simulink model "modeloSS_yama_LQI"  (R2016b)
settings: Solver=FixedStepDiscrete  StartTime=0.0  StopTime=20  FixedStep=0.001  RelTol=1e-3  EnableMultiTasking=on
values from neighbouring files (symbols this model uses):
  K_lqi = lqi(manolito,Q,R,N)    [marcelino_Lineal_LQI.m]
  Kb = 0.468    [Jacobian_marcelino.m]
  Kt = 0.317    [Jacobian_marcelino.m]    (also in Jacobian_marcelinoB.m)
  Rm = 6.69    [Jacobian_marcelino.m]    (also in Jacobian_marcelinoB.m)
undefined symbols (not defined in the file or in its folder): Cm, Cw, DiscIntNeverNeededParam, Jm, Jw, Lm, n
libraries: simulink x1
settings Model: Creator=FranRuzafa  LastModifiedBy=Miguel
settings OptimizationCC: LifeSpan=inf
settings DebuggingCC: SFUnexpectedBacktrackingDiag=warning  SFNoUnconditionalDefaultTransitionDiag=warning  SFExecutionAtInitializationDiag=none
settings GRTTargetCC: TargetLangStandard=C89/C90 (ANSI)  GeneratePreprocessorConditionals=Disable all
settings ConfigComp: CovMetricSettings=dw  CovHtmlReporting=on  CovSaveCumulativeToWorkspaceVar=on  CovSaveSingleToWorkspaceVar=on  CovExternalEMLEnable=off

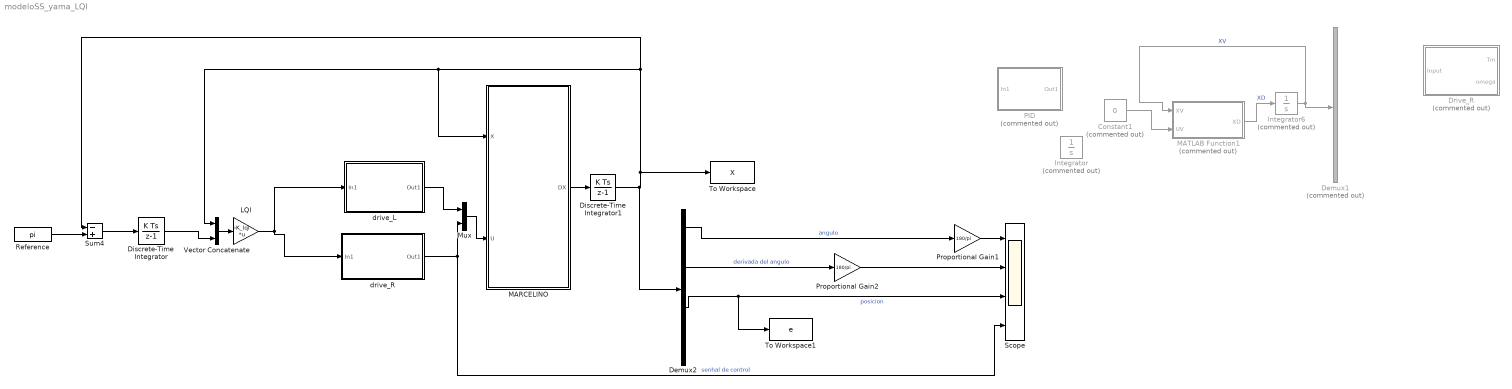
== system modeloSS_yama_LQI ==
  Constant1 : Constant  Commented=on  Value=0
  Demux1 : Demux  Commented=on
  Demux2 : Demux
  Discrete-Time Integrator : DiscreteIntegrator  InitialConditionSetting=State (most efficient)  SampleTime=-1  ICPrevOutput=DiscIntNeverNeededParam  ICPrevScaledInput=DiscIntNeverNeededParam
  Discrete-Time Integrator1 : DiscreteIntegrator  InitialCondition=[pi+0.2,0,0,0]  InitialConditionSetting=State (most efficient)  SampleTime=-1  ICPrevOutput=DiscIntNeverNeededParam  ICPrevScaledInput=DiscIntNeverNeededParam
  Drive_R : Subsystem  Commented=on
  Integrator : Integrator  Commented=on  InitialCondition=[pi+0.2,0,0,0]
  Integrator6 : Integrator  Commented=on  InitialCondition=[0;0;0.1;0]
  "LQI " : Gain  Gain=-K_lqi  Multiplication=Matrix(K*u)  SaturateOnIntegerOverflow=on  OutDataTypeStr=Inherit: Same as input  ParamDataTypeStr=Inherit: Same as input
  MARCELINO : MATLAB Function  TreatAsAtomicUnit=on
  MATLAB Function1 : MATLAB Function  Commented=on  TreatAsAtomicUnit=on
  Mux : Mux  Inputs=2
  PID : Subsystem  Commented=on
  Proportional Gain1 : Gain  Gain=180/pi  SaturateOnIntegerOverflow=on  OutDataTypeStr=Inherit: Same as input  ParamDataTypeStr=Inherit: Same as input
  Proportional Gain2 : Gain  Gain=180/pi  SaturateOnIntegerOverflow=on  OutDataTypeStr=Inherit: Same as input  ParamDataTypeStr=Inherit: Same as input
  Reference : Constant  Value=pi
  Scope : Scope  NumInputPorts=4
  Sum4 : Sum  Inputs=-+  SaturateOnIntegerOverflow=on  InputSameDT=on  OutDataTypeStr=Inherit: Same as first input
  To Workspace : ToWorkspace  VariableName=X  SampleTime=-1
      settings: Save2DSignal=2-D array (concatenate along first dimension)
  To Workspace1 : ToWorkspace  VariableName=e  SampleTime=-1
      settings: Save2DSignal=2-D array (concatenate along first dimension)
  Vector Concatenate : Concatenate
  drive_L : Subsystem
  "drive_R " : Subsystem
  wires:
  MARCELINO/1(DX) -> Discrete-Time Integrator1/1
  MATLAB Function1/1(XD) -> Integrator6/1  "XD"
  Integrator6/1 -> Demux1/1, MATLAB Function1/1(XV)  "XV"
  Constant1/1 -> MATLAB Function1/2(UV)
  Discrete-Time Integrator1/1 -> Demux2/1, Sum4/1, MARCELINO/1(X), Vector Concatenate/1, To Workspace/1
  Demux2/1 -> Proportional Gain1/1  "angulo"
  Reference/1 -> Sum4/2
  Proportional Gain1/1 -> Scope/1
  Sum4/1 -> Discrete-Time Integrator/1
  "drive_R "/1(Out1) -> Mux/2, Scope/4  "senhal de control"
  "LQI "/1 -> "drive_R "/1(In1), drive_L/1(In1)
  drive_L/1(Out1) -> Mux/1
  Mux/1 -> MARCELINO/2(U)
  Discrete-Time Integrator/1 -> Vector Concatenate/2
  Vector Concatenate/1 -> "LQI "/1
  Demux2/3 -> To Workspace1/1, Scope/3  "posicion"
  Demux2/2 -> Proportional Gain2/1  "derivada del angulo"
  Proportional Gain2/1 -> Scope/2

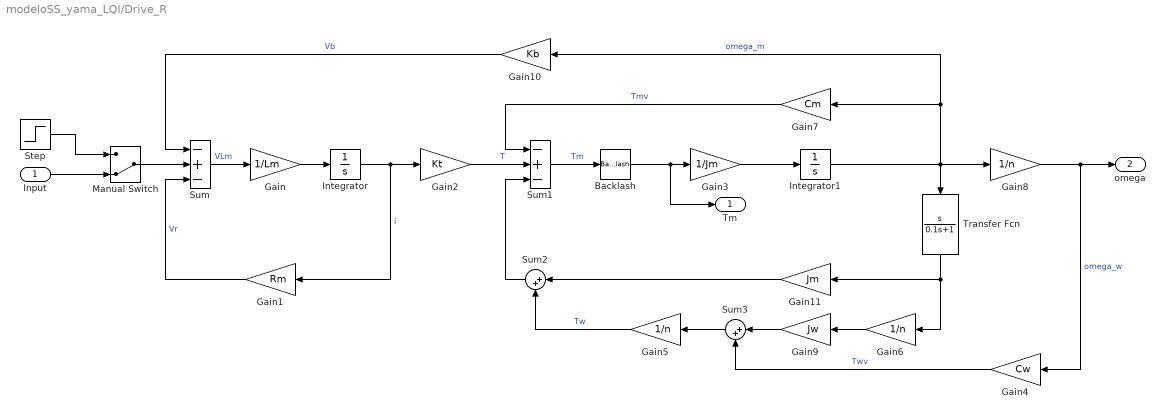
== system modeloSS_yama_LQI/Drive_R ==
  Input : Inport
  Backlash : Backlash  BacklashWidth=0.05
  Gain : Gain  Gain=1/Lm
  Gain1 : Gain  Gain=Rm
  Gain10 : Gain  Gain=Kb
  Gain11 : Gain  Gain=Jm
  Gain2 : Gain  Gain=Kt
  Gain3 : Gain  Gain=1/Jm
  Gain4 : Gain  Gain=Cw
  Gain5 : Gain  Gain=1/n
  Gain6 : Gain  Gain=1/n
  Gain7 : Gain  Gain=Cm
  Gain8 : Gain  Gain=1/n
  Gain9 : Gain  Gain=Jw
  Integrator : Integrator
  Integrator1 : Integrator
  Manual Switch : ManualSwitch  CurrentSetting=0
  Step : Step  After=9  SampleTime=0
  Sum : Sum  Inputs=-+-
  Sum1 : Sum  Inputs=-+-
  Sum2 : Sum  Inputs=|++
  Sum3 : Sum  Inputs=|++
  Transfer Fcn : TransferFcn  Numerator=[1 0]  Denominator=[0.1 1]
  Tm : Outport
  omega : Outport  Port=2
  wires:
  Sum/1 -> Gain/1  "VLm"
  Gain/1 -> Integrator/1
  Integrator/1 -> Gain2/1, Gain1/1  "i"
  Gain1/1 -> Sum/3  "Vr"
  Gain2/1 -> Sum1/2  "T"
  Sum1/1 -> Backlash/1  "Tm"
  Gain3/1 -> Integrator1/1
  Gain7/1 -> Sum1/1  "Tmv"
  Integrator1/1 -> Gain10/1, Gain7/1, Gain8/1, Transfer Fcn/1  "omega_m"
  Gain10/1 -> Sum/1  "Vb"
  Gain6/1 -> Gain9/1
  Sum3/1 -> Gain5/1
  Transfer Fcn/1 -> Gain6/1, Gain11/1
  Gain4/1 -> Sum3/2  "Twv"
  Gain9/1 -> Sum3/1
  Gain8/1 -> omega/1, Gain4/1  "omega_w"
  Manual Switch/1 -> Sum/2
  Input/1 -> Manual Switch/2
  Step/1 -> Manual Switch/1
  Sum2/1 -> Sum1/3
  Gain5/1 -> Sum2/2  "Tw"
  Gain11/1 -> Sum2/1
  Backlash/1 -> Gain3/1, Tm/1

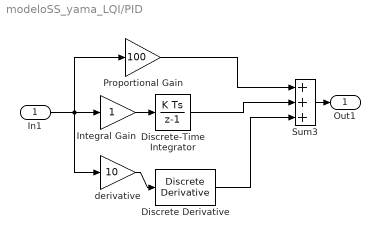
== system modeloSS_yama_LQI/PID ==
  In1 : Inport
  Discrete Derivative : simulink/Discrete/Discrete Derivative  gainval=1.0  ICPrevScaledInput=0.0  OutMin=[]  OutMax=[]  OutDataType=fixdt(1, 16)  OutScaling=2^-10  DoSatur=off
  Discrete-Time Integrator : DiscreteIntegrator  InitialConditionSetting=State (most efficient)  SampleTime=-1  ICPrevOutput=DiscIntNeverNeededParam  ICPrevScaledInput=DiscIntNeverNeededParam
  Integral Gain : Gain  SaturateOnIntegerOverflow=on  OutDataTypeStr=Inherit: Same as input  ParamDataTypeStr=Inherit: Same as input
  Proportional Gain : Gain  Gain=100  SaturateOnIntegerOverflow=on  OutDataTypeStr=Inherit: Same as input  ParamDataTypeStr=Inherit: Same as input
  Sum3 : Sum  Inputs=+++  SaturateOnIntegerOverflow=on  InputSameDT=on  OutDataTypeStr=Inherit: Same as first input
  "derivative " : Gain  Gain=10  SaturateOnIntegerOverflow=on  OutDataTypeStr=Inherit: Same as input  ParamDataTypeStr=Inherit: Same as input
  Out1 : Outport
  wires:
  "derivative "/1 -> Discrete Derivative/1
  Discrete Derivative/1 -> Sum3/3
  In1/1 -> "derivative "/1, Proportional Gain/1, Integral Gain/1
  Integral Gain/1 -> Discrete-Time Integrator/1
  Discrete-Time Integrator/1 -> Sum3/2
  Sum3/1 -> Out1/1
  Proportional Gain/1 -> Sum3/1

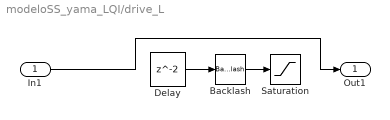
== system modeloSS_yama_LQI/drive_L ==
  In1 : Inport
  Backlash : Backlash  BacklashWidth=0.5
  Delay : Delay
  Saturation : Saturate  UpperLimit=15  LowerLimit=-15
  Out1 : Outport
  wires:
  In1/1 -> Out1/1
  Backlash/1 -> Saturation/1
  Delay/1 -> Backlash/1

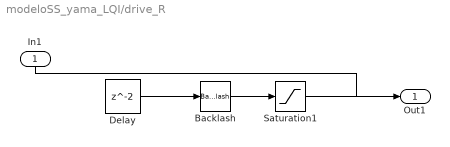
== system modeloSS_yama_LQI/drive_R  ==
  In1 : Inport
  Backlash : Backlash  BacklashWidth=0.5
  Delay : Delay
  Saturation1 : Saturate  UpperLimit=15  LowerLimit=-15
  Out1 : Outport
  wires:
  Delay/1 -> Backlash/1
  Saturation1/1 -> ?
  Backlash/1 -> Saturation1/1
  In1/1 -> Out1/1

== matlab function modeloSS_yama_LQI/MATLAB Function1 ==
  data: XV input; XD output; UV input
function XD = robotNL2( XV, UV )
%% robotNL
%   Modelo dinámico del robot. Ecuaciones del chino.
% XV = (theta, thetadot, Psi, Psidot, phi, phidot)
% UV = (vl, vr)

XD = zeros(4,1);
%vl = UV(1);
%vr = UV(2);
vl = UV;
vr = UV;

%% VALOR DE LOS PARÄMETROS DEL SISTEMA
g = 9.81;
m = 0.03;
R = 0.04;
Jw= m * R^2/2.0;
M = 0.6;
W = 0.14;
D = 0.04;
Hs = 0.144;
L = Hs/2.0;
JPsi = M*L^2 /3;
Jphi = M*(W^2 + D^2)/12.0;
Jm = 1E-5;
Rm = 6.69;
Kb = 0.468;
Kt = 0.317;
n = 1.0;
fm = 0.0022;
fw = 0.0;

%% MATRICES
alpha = (n*Kt)/(Rm);
beta = (n*Kt*Kb)/(Rm) + fm;

E = zeros(2);
E(1,1) = (2*m+M)*R^2 + 2*Jw + 2*n^2*Jm;
E(1,2) = M*L*R - 2*n^2*Jm;
E(2,1) = M*L*R - 2*n^2*Jm;
E(2,2) = M*L^2 + JPsi + 2*n^2*Jm;

F = zeros(2);
F(1,1) = beta + fw;
F(1,2) = -beta;
F(2,1) = -beta;
F(2,2) = beta;
F = 2*F;

G = zeros(2);
G(2,2) = -M*g*L;

H = zeros(2);
H(1,1) = alpha;
H(1,2) = alpha;
H(2,1) = -alpha;
H(2,2) = -alpha;

%I = (1/2)*m*W^2 + Jphi + (W^2)/(2*R^2)*(Jw + n^2*Jm);
%J = (W^2)/(2*R^2)*(beta + fw);
%K = (W)/(2*R) * alpha;

%% SISTEMA
% las ecuaciones son:
% E*(thetadot2; Psidot2) + F*(X2;X4) + G*(X1;X3) = H*(U1;U2)
% I*phidot2 + J*X6 = K* (U2-U1)

% despejar derivadas segundas
Einv = inv(E);

temp = -Einv*F*[XV(2);XV(4)] - Einv*G*[XV(1);XV(3)] + Einv*H*[vl;vr]; %#ok<MINV>

%% SALIDA
% thetadot
XD(1,1) = XV(2);
% thetadot2
XD(2,1) = temp(1);
% Psidot
XD(3,1) = XV(4);
% Psidot2
XD(4,1) = temp(2);
% % phidot
% XD(5,1) = XV(6);
% % phidot2
% XD(6,1) = K/I * (vl-vr) - J/I*XV(6);

end

== matlab function modeloSS_yama_LQI/MARCELINO ==
  data: DX output; X input; U input
function DX  = fcn(X,U)

g = 9.81; % gravedad
m = 0.03; % masa ruedas 
R = 0.028; % radio ruedas (0.056)
Jw = m * R^2/2.0; % Inercia ruedas
M = 60; % masa robot (con o sin ruedas, revisar) (0.63)
W = 0.09; % ancho robot sin ruedas (medir por si acaso)
D = 0.05; % Lo que sobresalen las ruedas 
%Hs = 0.26; % (0.315) HAY QUE MEDIR SIN RUEDA
L = 0.13; 
Jpsi = M*L^2 /3; % Momento de inercia eje ruedas
Jphi = M*(W^2 + D^2)/12.0; % Inercia del otro eje (¿Despreciable?)
Jm = 1E-5;
Rm = 6.69;
Kb = 0.468;
Kt = 0.317;
fm = 0.022;
fw = 0.0; % No se si debe despreciar
% x=X(3);
%%
l=0.13;
vl=U(1);
vr=U(2);
%%
F=(Kt/R*((((vl+vr))+Kb*(X(2)-(X(4)/R)))/Rm));
% F=(Kt/R*((V)/Rm));

% F=-0.05*sign(X(4));
%%
% F=V;
% X(1)=X(1)+0.1*sign(X(2));

DX=zeros(1,4);
DX(1)=X(2);
DX(2)=(F*cos(X(1))-(M+m)*g*sin(X(1))+m*l*(cos(X(1))*sin(X(1)))*X(2)^2)/(m*l*cos(X(1))^2-(M+m)*l);
DX(3)=X(4);
DX(4)=(F+m*l*(sin(X(1))*X(2)^2-m*g*cos(X(1))*sin(X(1))))/(M+m-m*cos(X(1))^2);
end
